simulink model "Ass2_extraA"  (R2024b)
settings: Solver=FixedStepAuto  StartTime=0.0  StopTime=inf  FixedStep=1/f_sim  RelTol=1e-3
values from neighbouring files (symbols this model uses):
  f_cmd = 100    [Main_ass2_extraA.m]
  f_odom = 100    [Main_ass2_extraA.m]
  f_waypoints = 100    [Main_ass2_extraA.m]
  K_dir = 10    [Main_ass2_extraA.m]
  K_dist = 1    [Main_ass2_extraA.m]
  K_or = 10    [Main_ass2_extraA.m]
  r = 0.05    [Main_ass2_extraA.m]
  toll_dist = 0.05    [Main_ass2_extraA.m]
  toll_orient = 0.03    [Main_ass2_extraA.m]
  v_max = 0.2    [Main_ass2_extraA.m]
  v_min = -0.2    [Main_ass2_extraA.m]
  w_max = 0.4    [Main_ass2_extraA.m]
  w_min = -0.4    [Main_ass2_extraA.m]
  waypoints = reshape(waypoints,[3 12])'    [Main_ass2_extraA.m]
undefined symbols (not defined in the file or in its folder): Angular, Linear
libraries: robotlib x4, simulink x3, hdlsllib x1
settings Model: Creator=vise  LastModifiedBy=vise
settings OptimizationCC: DefaultParameterBehavior=Inlined  EnhancedBackFolding=on  PassReuseOutputArgsAs=Individual arguments  ZeroExternalMemoryAtStartup=off  ZeroInternalMemoryAtStartup=off  MaxStackSize=64  OptimizeBlockOrder=speed  DifferentSizesBufferReuse=on  OptimizationCustomize=off  EfficientTunableParamExpr=on
settings DebuggingCC: ParameterTunabilityLossMsg=error
settings HardwareCC: ProdBitPerPointer=32  ProdBitPerSizeT=32  ProdBitPerPtrDiffT=32  ProdLargestAtomicFloat=None  ProdIntDivRoundTo=Undefined  ProdEndianess=Unspecified  ProdWordSize=32  ProdHWDeviceType=Generic->Unspecified (assume 32-bit Generic)  UseEmbeddedCoderFeatures=off
settings SFSimCC: MATLABDynamicMemAlloc=off
settings RTWCC: Description=Embedded Coder  SystemTargetFile=ert.tlc  HardwareBoard=Robot Operating System (ROS)  TLCOptions="-aInlineSetEventsForThisBaseRateFcn=TLC_FALSE -aSuppressMultiTaskScheduler=TLC_FALSE  -aRateBasedStepFcn=0"  TemplateMakefile=ert_default_tmf  Toolchain=Catkin  TargetLang=C++
settings CodeAppCC: ForceParamTrailComments=on  IgnoreCustomStorageClasses=off  OperatorAnnotations=on  SimulinkDataObjDesc=on  SFDataObjDesc=on  InsertBlockDesc=on
settings ERTTargetCC: SupportNonInlinedSFcns=on

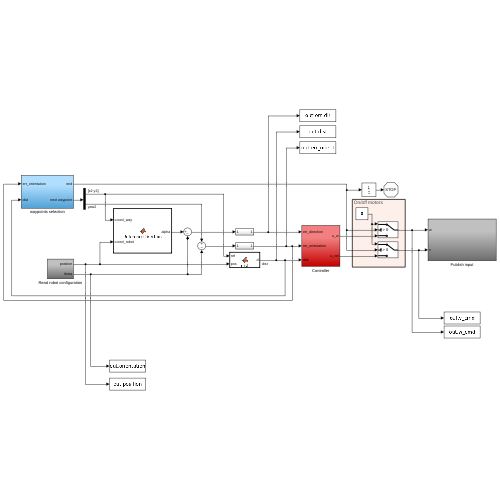
[thumbnail: Simulink's stored preview of the top-level diagram]
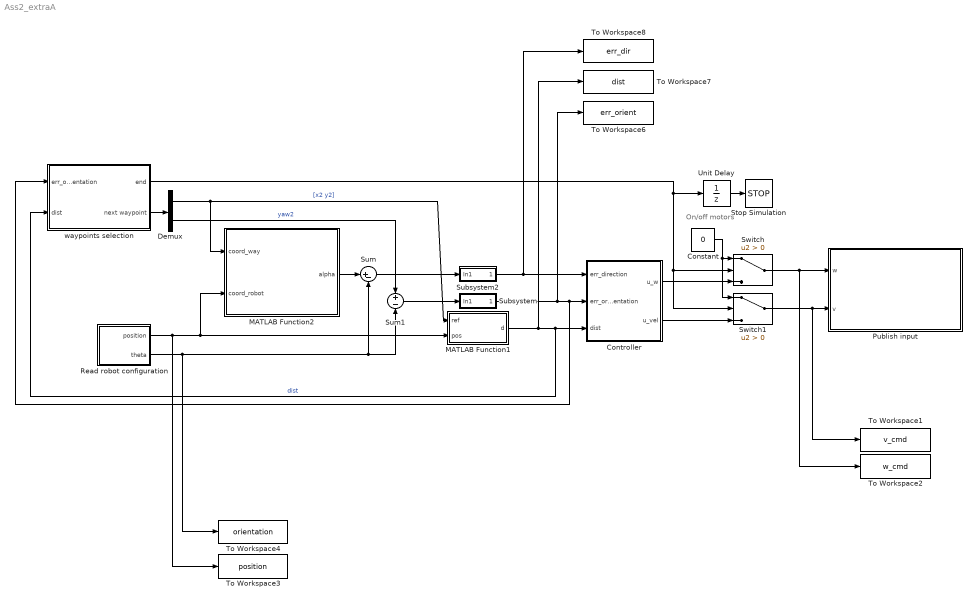
== system Ass2_extraA ==
  note: On/off motors
  Constant : Constant  Value=0
  Controller : Subsystem
  Demux : Demux  Outputs=2
  MATLAB Function1 : MATLAB Function  TreatAsAtomicUnit=on
  MATLAB Function2 : MATLAB Function  TreatAsAtomicUnit=on
  Publish input : Subsystem
  Read robot configuration : Subsystem
  Stop Simulation : Stop
  Subsystem : Subsystem
  Subsystem2 : Subsystem
  Sum : Sum  Inputs=|+-
  Sum1 : Sum  Inputs=+|-
  Switch : Switch  Criteria=u2 > Threshold  SaturateOnIntegerOverflow=off  InputSameDT=off
  Switch1 : Switch  Criteria=u2 > Threshold  SaturateOnIntegerOverflow=off  InputSameDT=off
  To Workspace1 : ToWorkspace  VariableName=v_cmd  SampleTime=-1
      settings: Save2DSignal=2-D array (concatenate along first dimension)
  To Workspace2 : ToWorkspace  VariableName=w_cmd  SampleTime=-1
      settings: Save2DSignal=2-D array (concatenate along first dimension)
  To Workspace3 : ToWorkspace  VariableName=position  SampleTime=-1
      settings: Save2DSignal=2-D array (concatenate along first dimension)
  To Workspace4 : ToWorkspace  VariableName=orientation  SampleTime=-1
      settings: Save2DSignal=2-D array (concatenate along first dimension)
  To Workspace6 : ToWorkspace  VariableName=err_orient  SampleTime=-1
      settings: Save2DSignal=2-D array (concatenate along first dimension)
  To Workspace7 : ToWorkspace  VariableName=dist  SampleTime=-1
      settings: Save2DSignal=2-D array (concatenate along first dimension)
  To Workspace8 : ToWorkspace  VariableName=err_dir  SampleTime=-1
      settings: Save2DSignal=2-D array (concatenate along first dimension)
  Unit Delay : UnitDelay  SampleTime=3  HasFrameUpgradeWarning=on
  waypoints selection : Subsystem
  wires:
  Demux/1 -> MATLAB Function2/1(coord_way), MATLAB Function1/1(ref)  "[x2 y2]"
  MATLAB Function1/1(d) -> Controller/3(dist), waypoints selection/2(dist), To Workspace7/1  "dist"
  MATLAB Function2/1(alpha) -> Sum/1
  Sum/1 -> Subsystem2/1(In1)
  Demux/2 -> Sum1/1  "yaw2"
  Sum1/1 -> Subsystem/1(In1)
  Read robot configuration/2(theta) -> Sum1/2, Sum/2, To Workspace4/1
  Controller/1(u_w) -> Switch/3
  Controller/2(u_vel) -> Switch1/3
  Switch/1 -> To Workspace2/1, Publish input/1(w)
  Switch1/1 -> To Workspace1/1, Publish input/2(v)
  Constant/1 -> Switch1/1, Switch/1
  Read robot configuration/1(position) -> MATLAB Function1/2(pos), MATLAB Function2/2(coord_robot), To Workspace3/1
  Subsystem2/1(Out1) -> To Workspace8/1, Controller/1(err_direction)
  Unit Delay/1 -> Stop Simulation/1
  Subsystem/1(Out1) -> waypoints selection/1(err_orientation), Controller/2(err_orientation), To Workspace6/1
  waypoints selection/1(end) -> Switch1/2, Switch/2, Unit Delay/1
  waypoints selection/2(next waypoint) -> Demux/1

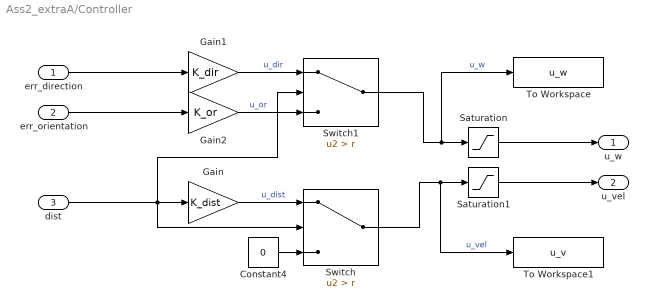
== system Ass2_extraA/Controller ==
  err_direction : Inport
  err_orientation : Inport  Port=2
  dist : Inport  Port=3
  Constant4 : Constant  Value=0
  Gain : Gain  Gain=K_dist
  Gain1 : Gain  Gain=K_dir
  Gain2 : Gain  Gain=K_or
  Saturation : Saturate  UpperLimit=w_max  LowerLimit=w_min
  Saturation1 : Saturate  UpperLimit=v_max  LowerLimit=v_min
  Switch : Switch  Criteria=u2 > Threshold  Threshold=r  SaturateOnIntegerOverflow=off  InputSameDT=off
  Switch1 : Switch  Criteria=u2 > Threshold  Threshold=r  SaturateOnIntegerOverflow=off  InputSameDT=off
  To Workspace : ToWorkspace  VariableName=u_w  SampleTime=-1
      settings: Save2DSignal=2-D array (concatenate along first dimension)
  To Workspace1 : ToWorkspace  VariableName=u_v  SampleTime=-1
      settings: Save2DSignal=2-D array (concatenate along first dimension)
  u_w : Outport
  u_vel : Outport  Port=2
  wires:
  Saturation/1 -> u_w/1
  err_orientation/1 -> Gain2/1
  err_direction/1 -> Gain1/1
  Switch1/1 -> To Workspace/1, Saturation/1  "u_w"
  Gain2/1 -> Switch1/3  "u_or"
  Constant4/1 -> Switch/3
  dist/1 -> Switch1/2, Switch/2, Gain/1
  Saturation1/1 -> u_vel/1
  Switch/1 -> To Workspace1/1, Saturation1/1  "u_vel"
  Gain/1 -> Switch/1  "u_dist"
  Gain1/1 -> Switch1/1  "u_dir"

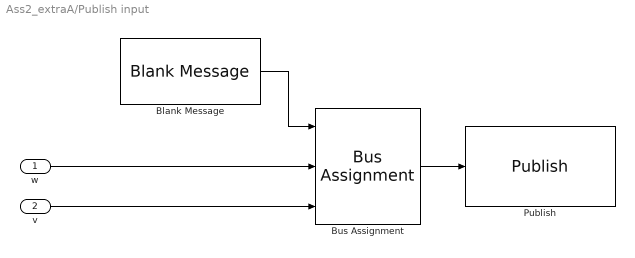
== system Ass2_extraA/Publish input ==
  w : Inport
  v : Inport  Port=2
  Blank Message : robotlib/Blank Message  messageClass=Message  entityType=geometry_msgs/Twist  messageType=geometry_msgs/Twist  SampleTime=1/f_cmd  legacyBusStruct=off
  Bus Assignment : BusAssignment  AssignedSignals=Angular.Z,Linear.X
  Publish : robotlib/Publish  topicSource=Select from ROS network  topic=/cmd_vel  messageType=geometry_msgs/Twist  legacyBusStruct=off  messageQueueLength=1
  wires:
  Bus Assignment/1 -> Publish/1
  Blank Message/1 -> Bus Assignment/1
  v/1 -> Bus Assignment/3
  w/1 -> Bus Assignment/2

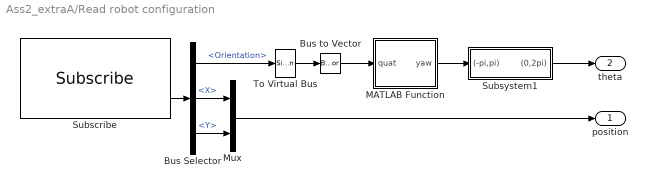
== system Ass2_extraA/Read robot configuration ==
  Bus Selector : BusSelector  OutputSignals=Pose.Pose.Orientation,Pose.Pose.Position.X,Pose.Pose.Position.Y
  Bus to Vector : BusToVector
  MATLAB Function : MATLAB Function  TreatAsAtomicUnit=on
  Mux : Mux  Inputs=2
  Subscribe : robotlib/Subscribe  topicSource=Select from ROS network  topic=/odom  messageType=nav_msgs/Odometry  SampleTime=1/f_odom  legacyBusStruct=off  messageQueueLength=1
  Subsystem1 : Subsystem
  To Virtual Bus : SignalConversion  ConversionOutput=Virtual bus  OverrideOpt=off
  position : Outport
  theta : Outport  Port=2
  wires:
  Bus to Vector/1 -> MATLAB Function/1(quat)
  Mux/1 -> position/1
  MATLAB Function/1(yaw) -> Subsystem1/1((-pi,pi))
  Bus Selector/1 -> To Virtual Bus/1  "<Orientation>"
  Bus Selector/2 -> Mux/1  "<X>"
  Subsystem1/1((0,2pi)) -> theta/1
  To Virtual Bus/1 -> Bus to Vector/1
  Subscribe/2 -> Bus Selector/1
  Bus Selector/3 -> Mux/2  "<Y>"

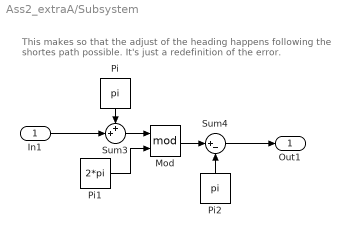
== system Ass2_extraA/Subsystem ==
  note: This makes so that the adjust of the heading happens following
      | the shortes path possible. It's just a redefinition of the error.
  In1 : Inport
  Mod : Math  Operator=mod
  Pi : Constant  Value=pi  OutDataTypeStr=Inherit: Inherit via back propagation
  Pi1 : Constant  Value=2*pi  OutDataTypeStr=Inherit: Inherit via back propagation
  Pi2 : Constant  Value=pi  OutDataTypeStr=Inherit: Inherit via back propagation
  Sum3 : Sum  Inputs=++|
  Sum4 : Sum  Inputs=|+-
  Out1 : Outport
  wires:
  Mod/1 -> Sum4/1
  Sum3/1 -> Mod/1
  Pi1/1 -> Mod/2
  Pi/1 -> Sum3/1
  Pi2/1 -> Sum4/2
  In1/1 -> Sum3/2
  Sum4/1 -> Out1/1

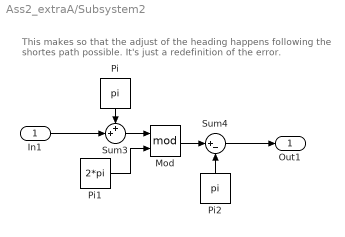
== system Ass2_extraA/Subsystem2 ==
  note: This makes so that the adjust of the heading happens following
      | the shortes path possible. It's just a redefinition of the error.
  In1 : Inport
  Mod : Math  Operator=mod
  Pi : Constant  Value=pi  OutDataTypeStr=Inherit: Inherit via back propagation
  Pi1 : Constant  Value=2*pi  OutDataTypeStr=Inherit: Inherit via back propagation
  Pi2 : Constant  Value=pi  OutDataTypeStr=Inherit: Inherit via back propagation
  Sum3 : Sum  Inputs=++|
  Sum4 : Sum  Inputs=|+-
  Out1 : Outport
  wires:
  Sum4/1 -> Out1/1
  In1/1 -> Sum3/2
  Pi2/1 -> Sum4/2
  Pi/1 -> Sum3/1
  Pi1/1 -> Mod/2
  Sum3/1 -> Mod/1
  Mod/1 -> Sum4/1

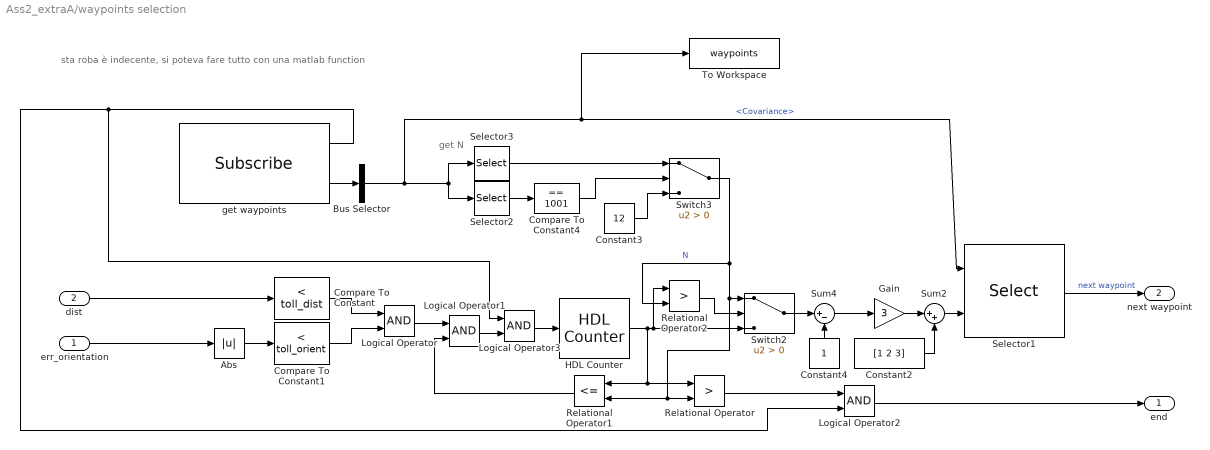
== system Ass2_extraA/waypoints selection ==
  note: sta roba è indecente, si poteva fare tutto con una matlab function
  note: get N
  err_orientation : Inport
  dist : Inport  Port=2
  Abs : Abs  SaturateOnIntegerOverflow=off
  Bus Selector : BusSelector  OutputSignals=Covariance
  Compare To Constant : simulink/Logic and Bit Operations/Compare To Constant  relop=<  const=toll_dist  OutDataTypeStr=boolean
  Compare To Constant1 : simulink/Logic and Bit Operations/Compare To Constant  relop=<  const=toll_orient  OutDataTypeStr=boolean
  Compare To Constant4 : simulink/Logic and Bit Operations/Compare To Constant  relop===  const=1001  OutDataTypeStr=boolean
  Constant2 : Constant  Value=[1 2 3]
  Constant3 : Constant  Value=12
  Constant4 : Constant
  Gain : Gain  Gain=3
  HDL Counter : hdlsllib/Sources/HDL Counter  CountType=Count limited  CountInit=1  CountStep=1  CountMax=13  CountFromType=Initial value  CountFrom=1  CountResetPort=off  CountLoadPort=off  CountEnbPort=on  CountDirPort=off  CountHitOutputPort=off  CountDataType=Unsigned  CountWordLen=8  CountFracLen=0  CountSampTime=1
  Logical Operator{,1..3} (4 alike) : Logic  AllPortsSameDT=off  OutDataTypeStr=boolean
  Relational Operator : RelationalOperator  Operator=>  OutDataTypeStr=boolean  RndMeth=Simplest  InputSameDT=off
  Relational Operator1 : RelationalOperator  Operator=<=  OutDataTypeStr=boolean  RndMeth=Simplest  InputSameDT=off
  Relational Operator2 : RelationalOperator  Operator=>  OutDataTypeStr=boolean  RndMeth=Simplest  InputSameDT=off
  Selector1 : Selector  InputPortWidth=36  IndexOptions=Index vector (port)  Indices=[1 3]  OutputSizes=1
  Selector2 : Selector  InputPortWidth=36  IndexOptions=Index vector (dialog)  Indices=35  OutputSizes=1
  Selector3 : Selector  InputPortWidth=36  IndexOptions=Index vector (dialog)  Indices=36  OutputSizes=1
  Sum2 : Sum  Inputs=|++
  Sum4 : Sum  Inputs=|+-
  Switch2 : Switch  Criteria=u2 > Threshold  SaturateOnIntegerOverflow=off  InputSameDT=off
  Switch3 : Switch  Criteria=u2 > Threshold  SaturateOnIntegerOverflow=off  InputSameDT=off
  To Workspace : ToWorkspace  VariableName=waypoints  SampleTime=-1
      settings: Save2DSignal=2-D array (concatenate along first dimension)
  get waypoints : robotlib/Subscribe  topicSource=Select from ROS network  topic=/waypoints  messageType=geometry_msgs/PoseWithCovariance  SampleTime=1/f_waypoints  legacyBusStruct=off  messageQueueLength=1
  end : Outport
  next waypoint : Outport  Port=2
  wires:
  Abs/1 -> Compare To Constant1/1
  err_orientation/1 -> Abs/1
  Constant2/1 -> Sum2/2
  Compare To Constant4/1 -> Switch3/2
  Relational Operator1/1 -> Logical Operator1/2
  Logical Operator/1 -> Logical Operator1/1
  get waypoints/2 -> Bus Selector/1
  Selector1/1 -> next waypoint/1  "next waypoint"
  Switch2/1 -> Sum4/1
  Constant4/1 -> Sum4/2
  Selector3/1 -> Switch3/1
  Switch3/1 -> Relational Operator2/2, Relational Operator1/2, Relational Operator/2, Switch2/1  "N"
  Compare To Constant1/1 -> Logical Operator/2
  Bus Selector/1 -> Selector2/1, Selector3/1, To Workspace/1, Selector1/1  "<Covariance>"
  Sum2/1 -> Selector1/2
  dist/1 -> Compare To Constant/1
  Gain/1 -> Sum2/1
  Relational Operator2/1 -> Switch2/2
  Constant3/1 -> Switch3/3
  HDL Counter/1 -> Relational Operator2/1, Switch2/3, Relational Operator1/1, Relational Operator/1
  Logical Operator2/1 -> end/1
  Sum4/1 -> Gain/1
  Compare To Constant/1 -> Logical Operator/1
  Selector2/1 -> Compare To Constant4/1
  get waypoints/1 -> Logical Operator3/1, Logical Operator2/2
  Relational Operator/1 -> Logical Operator2/1
  Logical Operator1/1 -> Logical Operator3/2
  Logical Operator3/1 -> HDL Counter/1

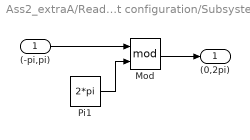
== system Ass2_extraA/Read robot configuration/Subsystem1 ==
  (-pi,pi) : Inport
  Mod : Math  Operator=mod
  Pi1 : Constant  Value=2*pi  OutDataTypeStr=Inherit: Inherit via back propagation
  (0,2pi) : Outport
  wires:
  (-pi,pi)/1 -> Mod/1
  Pi1/1 -> Mod/2
  Mod/1 -> (0,2pi)/1

== matlab function Ass2_extraA/Read robot configuration/MATLAB Function ==
  data: quat input; yaw output
function yaw=quat2yaw(quat)

q=zeros(1,4);

q(1)=quat(1);
q(2)=quat(2);
q(3)=quat(3);
q(4)=quat(4);

eul=quat2eul(q);

yaw=eul(3);

end

== matlab function Ass2_extraA/MATLAB Function2 ==
  data: coord_way input; alpha output; coord_robot input
function alpha=ReferenceDirection(coord_way,coord_robot)

% computes the direction (angle wrt positive x axis,
% counterclockwise) between two inputed points [x1 y1 ; x2 y2] 

x1=coord_robot(1);
y1=coord_robot(2);
x2=coord_way(1);
y2=coord_way(2);

alpha=atan2((y2-y1),(x2-x1)); % (-pi,pi)

alpha=mod(alpha,2*pi); % (0,2pi)

end

== matlab function Ass2_extraA/MATLAB Function1 ==
  data: ref input; d output; pos input
function d=dist(ref,pos)

% computes the distance between two points (x1,y1) and (x2,y2)

x_ref=ref(1);
y_ref=ref(2);
x_pos=pos(1);
y_pos=pos(2);

d=sqrt((x_ref-x_pos)^2+(y_ref-y_pos)^2);

end
